simulink subsystem "INA219_Voltage_Sensor"  (R2022b)
settings: Solver=VariableStepAuto  StartTime=0.0  StopTime=10.0  RelTol=1e-3
libraries: simulink x2
settings Model: Creator=gotta  LastModifiedBy=gotta

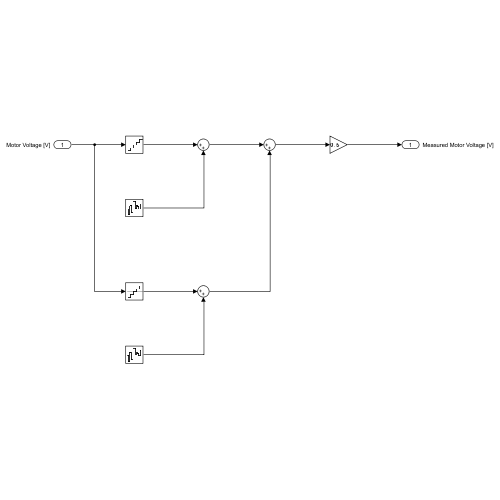
[thumbnail: Simulink's stored preview of the top-level diagram]
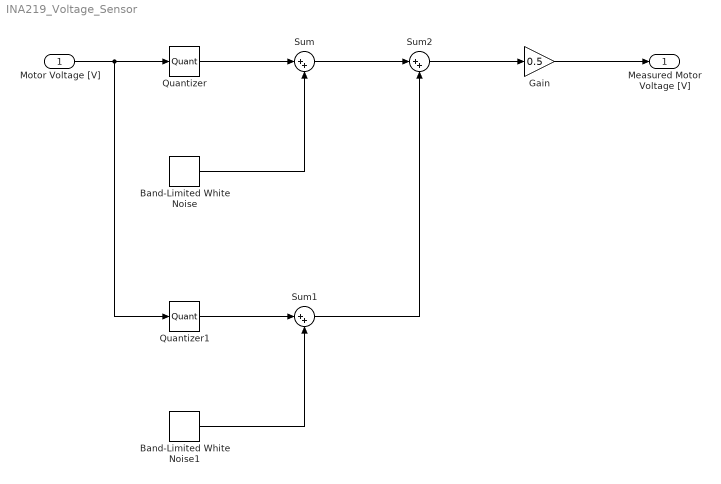
== system INA219_Voltage_Sensor ==
  Motor Voltage [V] : Inport
  Band-Limited White Noise : simulink/Sources/Band-Limited White Noise  Cov=[1e-6]  Ts=1e-3  seed=[23341]
  Band-Limited White Noise1 : simulink/Sources/Band-Limited White Noise  Cov=[1e-6]  Ts=1e-3  seed=[24560]
  Gain : Gain  Gain=0.5
  Quantizer : Quantizer  QuantizationInterval=INA219.voltage_LSB
  Quantizer1 : Quantizer  QuantizationInterval=INA219.voltage_LSB
  Sum : Sum  Inputs=|++
  Sum1 : Sum  Inputs=|++
  Sum2 : Sum  Inputs=|++
  Measured Motor Voltage [V] : Outport
  wires:
  Gain/1 -> Measured Motor Voltage [V]/1
  Quantizer1/1 -> Sum1/1
  Motor Voltage [V]/1 -> Quantizer1/1, Quantizer/1
  Band-Limited White Noise1/1 -> Sum1/2
  Sum/1 -> Sum2/1
  Sum2/1 -> Gain/1
  Sum1/1 -> Sum2/2
  Quantizer/1 -> Sum/1
  Band-Limited White Noise/1 -> Sum/2
